simulink model "COSTEP_Exergy"  (R2024b)
settings: Solver=FixedStepAuto  StartTime=0.0  StopTime=25  FixedStep=1/3600  RelTol=1e-3
model workspace (MAT data in the model file):
  AD : Simulink.Parameter (value not decoded)
  AG : Simulink.Parameter (value not decoded)
  AH : Simulink.Parameter (value not decoded)
  AV : Simulink.Parameter (value not decoded)
  AVP : Simulink.Parameter (value not decoded)
  BCHL : Simulink.Parameter (value not decoded)
  BCHV : Simulink.Parameter (value not decoded)
  BD : Simulink.Parameter (value not decoded)
  BDIST : Simulink.Parameter (value not decoded)
  BG : Simulink.Parameter (value not decoded)
  BH : Simulink.Parameter (value not decoded)
  BVP : Simulink.Parameter (value not decoded)
  CD : Simulink.Parameter (value not decoded)
  CDIST : Simulink.Parameter (value not decoded)
  CG : Simulink.Parameter (value not decoded)
  CH : Simulink.Parameter (value not decoded)
  CVP : Simulink.Parameter (value not decoded)
  DDIST : Simulink.Parameter (value not decoded)
  DIST_CONST : Simulink.Parameter (value not decoded)
  ISV : Simulink.Parameter (value not decoded)
  TLAST : Simulink.Parameter (value not decoded)
  TNEXT : Simulink.Parameter (value not decoded)
  XMW : Simulink.Parameter (value not decoded)
  XNS : Simulink.Parameter (value not decoded)
  XNS2 : Simulink.Parameter (value not decoded)
  XNS3 : Simulink.Parameter (value not decoded)
  XNSADD : Simulink.Parameter (value not decoded)
  XNSE : Simulink.Parameter (value not decoded)
symbols that are objects in the model workspace (value not decoded): AD, AG, AH, AV, AVP, BD, BG, BH, BVP, CD, CG, CH, CVP, XMW, XNS, XNS2, XNS3, XNSE
undefined symbols (not defined in the file or in its folder): magnitude, msgbox, SETPT, XMEAS, XMV
libraries: mylib x403, dspindex x31
(part 13 of 13)

== system COSTEP_Exergy/Random number generator/Stream Measurements SMEAS Gas analysis1/If Action Subsystem3/Subsystem/Stream 5/Subsystem/TESUB6 XMNSEE ==
  G : Inport
  Process Noise I=1-12 G New : mylib/Process Noise I=1-12 G New  SystemSampleTime=-1  VariantActivationTime=update diagram  AllowFlexibleInterface=on  Latency=0  AutoFrameSizeCalculation=off
  XNSEE : Constant  Value=0.25
  XMNSEE : Outport  VectorParamsAs1DForOutWhenUnconnected=off
  G_NEW : Outport  Port=2  VectorParamsAs1DForOutWhenUnconnected=off
  wires:
  XNSEE/1 -> Process Noise I=1-12 G New/1
  Process Noise I=1-12 G New/1 -> XMNSEE/1
  G/1 -> Process Noise I=1-12 G New/2
  Process Noise I=1-12 G New/2 -> G_NEW/1

== system COSTEP_Exergy/Random number generator/Stream Measurements SMEAS Gas analysis1/If Action Subsystem3/Subsystem/Stream 5/Subsystem/TESUB6 XMNSEF ==
  G : Inport
  Process Noise I=1-12 G New : mylib/Process Noise I=1-12 G New  SystemSampleTime=-1  VariantActivationTime=update diagram  AllowFlexibleInterface=on  Latency=0  AutoFrameSizeCalculation=off
  XNSEF : Constant  Value=0.025
  XMNSEF : Outport  VectorParamsAs1DForOutWhenUnconnected=off
  G_NEW : Outport  Port=2  VectorParamsAs1DForOutWhenUnconnected=off
  wires:
  XNSEF/1 -> Process Noise I=1-12 G New/1
  Process Noise I=1-12 G New/1 -> XMNSEF/1
  G/1 -> Process Noise I=1-12 G New/2
  Process Noise I=1-12 G New/2 -> G_NEW/1

== system COSTEP_Exergy/Random number generator/Stream Measurements SMEAS Gas analysis1/If Action Subsystem3/Subsystem/Stream 5/Subsystem/TESUB6 XMNSEG ==
  G : Inport
  Process Noise I=1-12 G New : mylib/Process Noise I=1-12 G New  SystemSampleTime=-1  VariantActivationTime=update diagram  AllowFlexibleInterface=on  Latency=0  AutoFrameSizeCalculation=off
  XNSEG : Constant  Value=0.05
  XMNSEG : Outport  VectorParamsAs1DForOutWhenUnconnected=off
  G_NEW : Outport  Port=2  VectorParamsAs1DForOutWhenUnconnected=off
  wires:
  XNSEG/1 -> Process Noise I=1-12 G New/1
  Process Noise I=1-12 G New/1 -> XMNSEG/1
  G/1 -> Process Noise I=1-12 G New/2
  Process Noise I=1-12 G New/2 -> G_NEW/1

== system COSTEP_Exergy/Random number generator/Stream Measurements SMEAS Gas analysis1/If Action Subsystem3/Subsystem/Stream 5/Subsystem/TESUB6 XMNSEH ==
  G : Inport
  Process Noise I=1-12 G New : mylib/Process Noise I=1-12 G New  SystemSampleTime=-1  VariantActivationTime=update diagram  AllowFlexibleInterface=on  Latency=0  AutoFrameSizeCalculation=off
  XNSEH : Constant  Value=0.05
  XMNSEH : Outport  VectorParamsAs1DForOutWhenUnconnected=off
  G_NEW : Outport  Port=2  VectorParamsAs1DForOutWhenUnconnected=off
  wires:
  XNSEH/1 -> Process Noise I=1-12 G New/1
  Process Noise I=1-12 G New/1 -> XMNSEH/1
  G/1 -> Process Noise I=1-12 G New/2
  Process Noise I=1-12 G New/2 -> G_NEW/1

== system COSTEP_Exergy/Random number generator/Stream Measurements SMEAS Gas analysis1/If Action Subsystem3/Subsystem/Stream 6/Subsystem/TESUB6 XMNSEA ==
  G : Inport
  Process Noise I=1-12 G New : mylib/Process Noise I=1-12 G New  SystemSampleTime=-1  VariantActivationTime=update diagram  AllowFlexibleInterface=on  Latency=0  AutoFrameSizeCalculation=off
  XNSEA : Constant  Value=0.25
  XMNSEA : Outport  VectorParamsAs1DForOutWhenUnconnected=off
  G_NEW : Outport  Port=2  VectorParamsAs1DForOutWhenUnconnected=off
  wires:
  XNSEA/1 -> Process Noise I=1-12 G New/1
  Process Noise I=1-12 G New/1 -> XMNSEA/1
  G/1 -> Process Noise I=1-12 G New/2
  Process Noise I=1-12 G New/2 -> G_NEW/1

== system COSTEP_Exergy/Random number generator/Stream Measurements SMEAS Gas analysis1/If Action Subsystem3/Subsystem/Stream 6/Subsystem/TESUB6 XMNSEB ==
  G : Inport
  Process Noise I=1-12 G New : mylib/Process Noise I=1-12 G New  SystemSampleTime=-1  VariantActivationTime=update diagram  AllowFlexibleInterface=on  Latency=0  AutoFrameSizeCalculation=off
  XNSEB : Constant  Value=0.1
  XMNSEB : Outport  VectorParamsAs1DForOutWhenUnconnected=off
  G_NEW : Outport  Port=2  VectorParamsAs1DForOutWhenUnconnected=off
  wires:
  XNSEB/1 -> Process Noise I=1-12 G New/1
  Process Noise I=1-12 G New/1 -> XMNSEB/1
  G/1 -> Process Noise I=1-12 G New/2
  Process Noise I=1-12 G New/2 -> G_NEW/1

== system COSTEP_Exergy/Random number generator/Stream Measurements SMEAS Gas analysis1/If Action Subsystem3/Subsystem/Stream 6/Subsystem/TESUB6 XMNSEC ==
  G : Inport
  Process Noise I=1-12 G New : mylib/Process Noise I=1-12 G New  SystemSampleTime=-1  VariantActivationTime=update diagram  AllowFlexibleInterface=on  Latency=0  AutoFrameSizeCalculation=off
  XNSEC : Constant  Value=0.25
  XMNSEC : Outport  VectorParamsAs1DForOutWhenUnconnected=off
  G_NEW : Outport  Port=2  VectorParamsAs1DForOutWhenUnconnected=off
  wires:
  XNSEC/1 -> Process Noise I=1-12 G New/1
  Process Noise I=1-12 G New/1 -> XMNSEC/1
  G/1 -> Process Noise I=1-12 G New/2
  Process Noise I=1-12 G New/2 -> G_NEW/1

== system COSTEP_Exergy/Random number generator/Stream Measurements SMEAS Gas analysis1/If Action Subsystem3/Subsystem/Stream 6/Subsystem/TESUB6 XMNSED ==
  G : Inport
  Process Noise I=1-12 G New : mylib/Process Noise I=1-12 G New  SystemSampleTime=-1  VariantActivationTime=update diagram  AllowFlexibleInterface=on  Latency=0  AutoFrameSizeCalculation=off
  XNSED : Constant  Value=0.1
  XMNSED : Outport  VectorParamsAs1DForOutWhenUnconnected=off
  G_NEW : Outport  Port=2  VectorParamsAs1DForOutWhenUnconnected=off
  wires:
  XNSED/1 -> Process Noise I=1-12 G New/1
  Process Noise I=1-12 G New/1 -> XMNSED/1
  G/1 -> Process Noise I=1-12 G New/2
  Process Noise I=1-12 G New/2 -> G_NEW/1

== system COSTEP_Exergy/Random number generator/Stream Measurements SMEAS Gas analysis1/If Action Subsystem3/Subsystem/Stream 6/Subsystem/TESUB6 XMNSEE ==
  G : Inport
  Process Noise I=1-12 G New : mylib/Process Noise I=1-12 G New  SystemSampleTime=-1  VariantActivationTime=update diagram  AllowFlexibleInterface=on  Latency=0  AutoFrameSizeCalculation=off
  XNSEE : Constant  Value=0.25
  XMNSEE : Outport  VectorParamsAs1DForOutWhenUnconnected=off
  G_NEW : Outport  Port=2  VectorParamsAs1DForOutWhenUnconnected=off
  wires:
  XNSEE/1 -> Process Noise I=1-12 G New/1
  Process Noise I=1-12 G New/1 -> XMNSEE/1
  G/1 -> Process Noise I=1-12 G New/2
  Process Noise I=1-12 G New/2 -> G_NEW/1

== system COSTEP_Exergy/Random number generator/Stream Measurements SMEAS Gas analysis1/If Action Subsystem3/Subsystem/Stream 6/Subsystem/TESUB6 XMNSEF ==
  G : Inport
  Process Noise I=1-12 G New : mylib/Process Noise I=1-12 G New  SystemSampleTime=-1  VariantActivationTime=update diagram  AllowFlexibleInterface=on  Latency=0  AutoFrameSizeCalculation=off
  XNSEF : Constant  Value=0.025
  XMNSEF : Outport  VectorParamsAs1DForOutWhenUnconnected=off
  G_NEW : Outport  Port=2  VectorParamsAs1DForOutWhenUnconnected=off
  wires:
  XNSEF/1 -> Process Noise I=1-12 G New/1
  Process Noise I=1-12 G New/1 -> XMNSEF/1
  G/1 -> Process Noise I=1-12 G New/2
  Process Noise I=1-12 G New/2 -> G_NEW/1

== system COSTEP_Exergy/Random number generator/Stream Measurements SMEAS Gas analysis1/If Action Subsystem3/Subsystem/Stream 6/Subsystem/TESUB6 XMNSEG ==
  G : Inport
  Process Noise I=1-12 G New : mylib/Process Noise I=1-12 G New  SystemSampleTime=-1  VariantActivationTime=update diagram  AllowFlexibleInterface=on  Latency=0  AutoFrameSizeCalculation=off
  XNSEG : Constant  Value=0.05
  XMNSEG : Outport  VectorParamsAs1DForOutWhenUnconnected=off
  G_NEW : Outport  Port=2  VectorParamsAs1DForOutWhenUnconnected=off
  wires:
  XNSEG/1 -> Process Noise I=1-12 G New/1
  Process Noise I=1-12 G New/1 -> XMNSEG/1
  G/1 -> Process Noise I=1-12 G New/2
  Process Noise I=1-12 G New/2 -> G_NEW/1

== system COSTEP_Exergy/Random number generator/Stream Measurements SMEAS Gas analysis1/If Action Subsystem3/Subsystem/Stream 6/Subsystem/TESUB6 XMNSEH ==
  G : Inport
  Process Noise I=1-12 G New : mylib/Process Noise I=1-12 G New  SystemSampleTime=-1  VariantActivationTime=update diagram  AllowFlexibleInterface=on  Latency=0  AutoFrameSizeCalculation=off
  XNSEH : Constant  Value=0.05
  XMNSEH : Outport  VectorParamsAs1DForOutWhenUnconnected=off
  G_NEW : Outport  Port=2  VectorParamsAs1DForOutWhenUnconnected=off
  wires:
  XNSEH/1 -> Process Noise I=1-12 G New/1
  Process Noise I=1-12 G New/1 -> XMNSEH/1
  G/1 -> Process Noise I=1-12 G New/2
  Process Noise I=1-12 G New/2 -> G_NEW/1

== system COSTEP_Exergy/Random number generator/Stream Measurements SMEAS Gas analysis1/If Action Subsystem3/Subsystem/Stream 8/Subsystem/TESUB6 XMNSEA ==
  G : Inport
  Process Noise I=1-12 G New : mylib/Process Noise I=1-12 G New  SystemSampleTime=-1  VariantActivationTime=update diagram  AllowFlexibleInterface=on  Latency=0  AutoFrameSizeCalculation=off
  XNSEA : Constant  Value=0.25
  XMNSEA : Outport  VectorParamsAs1DForOutWhenUnconnected=off
  G_NEW : Outport  Port=2  VectorParamsAs1DForOutWhenUnconnected=off
  wires:
  XNSEA/1 -> Process Noise I=1-12 G New/1
  Process Noise I=1-12 G New/1 -> XMNSEA/1
  G/1 -> Process Noise I=1-12 G New/2
  Process Noise I=1-12 G New/2 -> G_NEW/1

== system COSTEP_Exergy/Random number generator/Stream Measurements SMEAS Gas analysis1/If Action Subsystem3/Subsystem/Stream 8/Subsystem/TESUB6 XMNSEB ==
  G : Inport
  Process Noise I=1-12 G New : mylib/Process Noise I=1-12 G New  SystemSampleTime=-1  VariantActivationTime=update diagram  AllowFlexibleInterface=on  Latency=0  AutoFrameSizeCalculation=off
  XNSEB : Constant  Value=0.1
  XMNSEB : Outport  VectorParamsAs1DForOutWhenUnconnected=off
  G_NEW : Outport  Port=2  VectorParamsAs1DForOutWhenUnconnected=off
  wires:
  XNSEB/1 -> Process Noise I=1-12 G New/1
  Process Noise I=1-12 G New/1 -> XMNSEB/1
  G/1 -> Process Noise I=1-12 G New/2
  Process Noise I=1-12 G New/2 -> G_NEW/1

== system COSTEP_Exergy/Random number generator/Stream Measurements SMEAS Gas analysis1/If Action Subsystem3/Subsystem/Stream 8/Subsystem/TESUB6 XMNSEC ==
  G : Inport
  Process Noise I=1-12 G New : mylib/Process Noise I=1-12 G New  SystemSampleTime=-1  VariantActivationTime=update diagram  AllowFlexibleInterface=on  Latency=0  AutoFrameSizeCalculation=off
  XNSEC : Constant  Value=0.25
  XMNSEC : Outport  VectorParamsAs1DForOutWhenUnconnected=off
  G_NEW : Outport  Port=2  VectorParamsAs1DForOutWhenUnconnected=off
  wires:
  XNSEC/1 -> Process Noise I=1-12 G New/1
  Process Noise I=1-12 G New/1 -> XMNSEC/1
  G/1 -> Process Noise I=1-12 G New/2
  Process Noise I=1-12 G New/2 -> G_NEW/1

== system COSTEP_Exergy/Random number generator/Stream Measurements SMEAS Gas analysis1/If Action Subsystem3/Subsystem/Stream 8/Subsystem/TESUB6 XMNSED ==
  G : Inport
  Process Noise I=1-12 G New : mylib/Process Noise I=1-12 G New  SystemSampleTime=-1  VariantActivationTime=update diagram  AllowFlexibleInterface=on  Latency=0  AutoFrameSizeCalculation=off
  XNSED : Constant  Value=0.1
  XMNSED : Outport  VectorParamsAs1DForOutWhenUnconnected=off
  G_NEW : Outport  Port=2  VectorParamsAs1DForOutWhenUnconnected=off
  wires:
  XNSED/1 -> Process Noise I=1-12 G New/1
  Process Noise I=1-12 G New/1 -> XMNSED/1
  G/1 -> Process Noise I=1-12 G New/2
  Process Noise I=1-12 G New/2 -> G_NEW/1

== system COSTEP_Exergy/Random number generator/Stream Measurements SMEAS Gas analysis1/If Action Subsystem3/Subsystem/Stream 8/Subsystem/TESUB6 XMNSEE ==
  G : Inport
  Process Noise I=1-12 G New : mylib/Process Noise I=1-12 G New  SystemSampleTime=-1  VariantActivationTime=update diagram  AllowFlexibleInterface=on  Latency=0  AutoFrameSizeCalculation=off
  XNSEE : Constant  Value=0.25
  XMNSEE : Outport  VectorParamsAs1DForOutWhenUnconnected=off
  G_NEW : Outport  Port=2  VectorParamsAs1DForOutWhenUnconnected=off
  wires:
  XNSEE/1 -> Process Noise I=1-12 G New/1
  Process Noise I=1-12 G New/1 -> XMNSEE/1
  G/1 -> Process Noise I=1-12 G New/2
  Process Noise I=1-12 G New/2 -> G_NEW/1

== system COSTEP_Exergy/Random number generator/Stream Measurements SMEAS Gas analysis1/If Action Subsystem3/Subsystem/Stream 8/Subsystem/TESUB6 XMNSEF ==
  G : Inport
  Process Noise I=1-12 G New : mylib/Process Noise I=1-12 G New  SystemSampleTime=-1  VariantActivationTime=update diagram  AllowFlexibleInterface=on  Latency=0  AutoFrameSizeCalculation=off
  XNSEF : Constant  Value=0.025
  XMNSEF : Outport  VectorParamsAs1DForOutWhenUnconnected=off
  G_NEW : Outport  Port=2  VectorParamsAs1DForOutWhenUnconnected=off
  wires:
  XNSEF/1 -> Process Noise I=1-12 G New/1
  Process Noise I=1-12 G New/1 -> XMNSEF/1
  G/1 -> Process Noise I=1-12 G New/2
  Process Noise I=1-12 G New/2 -> G_NEW/1

== system COSTEP_Exergy/Random number generator/Stream Measurements SMEAS Gas analysis1/If Action Subsystem3/Subsystem/Stream 8/Subsystem/TESUB6 XMNSEG ==
  G : Inport
  Process Noise I=1-12 G New : mylib/Process Noise I=1-12 G New  SystemSampleTime=-1  VariantActivationTime=update diagram  AllowFlexibleInterface=on  Latency=0  AutoFrameSizeCalculation=off
  XNSEG : Constant  Value=0.05
  XMNSEG : Outport  VectorParamsAs1DForOutWhenUnconnected=off
  G_NEW : Outport  Port=2  VectorParamsAs1DForOutWhenUnconnected=off
  wires:
  XNSEG/1 -> Process Noise I=1-12 G New/1
  Process Noise I=1-12 G New/1 -> XMNSEG/1
  G/1 -> Process Noise I=1-12 G New/2
  Process Noise I=1-12 G New/2 -> G_NEW/1

== system COSTEP_Exergy/Random number generator/Stream Measurements SMEAS Gas analysis1/If Action Subsystem3/Subsystem/Stream 8/Subsystem/TESUB6 XMNSEH ==
  G : Inport
  Process Noise I=1-12 G New : mylib/Process Noise I=1-12 G New  SystemSampleTime=-1  VariantActivationTime=update diagram  AllowFlexibleInterface=on  Latency=0  AutoFrameSizeCalculation=off
  XNSEH : Constant  Value=0.05
  XMNSEH : Outport  VectorParamsAs1DForOutWhenUnconnected=off
  G_NEW : Outport  Port=2  VectorParamsAs1DForOutWhenUnconnected=off
  wires:
  XNSEH/1 -> Process Noise I=1-12 G New/1
  Process Noise I=1-12 G New/1 -> XMNSEH/1
  G/1 -> Process Noise I=1-12 G New/2
  Process Noise I=1-12 G New/2 -> G_NEW/1

== system COSTEP_Exergy/Random number generator/Stream Measurements SMEAS Gas analysis1/If Action Subsystem3/Subsystem/Stream 9/Subsystem/TESUB6 XMNSEA ==
  G : Inport
  Process Noise I=1-12 G New : mylib/Process Noise I=1-12 G New  SystemSampleTime=-1  VariantActivationTime=update diagram  AllowFlexibleInterface=on  Latency=0  AutoFrameSizeCalculation=off
  XNSEA : Constant  Value=0.25
  XMNSEA : Outport  VectorParamsAs1DForOutWhenUnconnected=off
  G_NEW : Outport  Port=2  VectorParamsAs1DForOutWhenUnconnected=off
  wires:
  XNSEA/1 -> Process Noise I=1-12 G New/1
  Process Noise I=1-12 G New/1 -> XMNSEA/1
  G/1 -> Process Noise I=1-12 G New/2
  Process Noise I=1-12 G New/2 -> G_NEW/1

== system COSTEP_Exergy/Random number generator/Stream Measurements SMEAS Gas analysis1/If Action Subsystem3/Subsystem/Stream 9/Subsystem/TESUB6 XMNSEB ==
  G : Inport
  Process Noise I=1-12 G New : mylib/Process Noise I=1-12 G New  SystemSampleTime=-1  VariantActivationTime=update diagram  AllowFlexibleInterface=on  Latency=0  AutoFrameSizeCalculation=off
  XNSEB : Constant  Value=0.1
  XMNSEB : Outport  VectorParamsAs1DForOutWhenUnconnected=off
  G_NEW : Outport  Port=2  VectorParamsAs1DForOutWhenUnconnected=off
  wires:
  XNSEB/1 -> Process Noise I=1-12 G New/1
  Process Noise I=1-12 G New/1 -> XMNSEB/1
  G/1 -> Process Noise I=1-12 G New/2
  Process Noise I=1-12 G New/2 -> G_NEW/1

== system COSTEP_Exergy/Random number generator/Stream Measurements SMEAS Gas analysis1/If Action Subsystem3/Subsystem/Stream 9/Subsystem/TESUB6 XMNSEC ==
  G : Inport
  Process Noise I=1-12 G New : mylib/Process Noise I=1-12 G New  SystemSampleTime=-1  VariantActivationTime=update diagram  AllowFlexibleInterface=on  Latency=0  AutoFrameSizeCalculation=off
  XNSEC : Constant  Value=0.25
  XMNSEC : Outport  VectorParamsAs1DForOutWhenUnconnected=off
  G_NEW : Outport  Port=2  VectorParamsAs1DForOutWhenUnconnected=off
  wires:
  XNSEC/1 -> Process Noise I=1-12 G New/1
  Process Noise I=1-12 G New/1 -> XMNSEC/1
  G/1 -> Process Noise I=1-12 G New/2
  Process Noise I=1-12 G New/2 -> G_NEW/1

== system COSTEP_Exergy/Random number generator/Stream Measurements SMEAS Gas analysis1/If Action Subsystem3/Subsystem/Stream 9/Subsystem/TESUB6 XMNSED ==
  G : Inport
  Process Noise I=1-12 G New : mylib/Process Noise I=1-12 G New  SystemSampleTime=-1  VariantActivationTime=update diagram  AllowFlexibleInterface=on  Latency=0  AutoFrameSizeCalculation=off
  XNSED : Constant  Value=0.1
  XMNSED : Outport  VectorParamsAs1DForOutWhenUnconnected=off
  G_NEW : Outport  Port=2  VectorParamsAs1DForOutWhenUnconnected=off
  wires:
  XNSED/1 -> Process Noise I=1-12 G New/1
  Process Noise I=1-12 G New/1 -> XMNSED/1
  G/1 -> Process Noise I=1-12 G New/2
  Process Noise I=1-12 G New/2 -> G_NEW/1

== system COSTEP_Exergy/Random number generator/Stream Measurements SMEAS Gas analysis1/If Action Subsystem3/Subsystem/Stream 9/Subsystem/TESUB6 XMNSEE ==
  G : Inport
  Process Noise I=1-12 G New : mylib/Process Noise I=1-12 G New  SystemSampleTime=-1  VariantActivationTime=update diagram  AllowFlexibleInterface=on  Latency=0  AutoFrameSizeCalculation=off
  XNSEE : Constant  Value=0.25
  XMNSEE : Outport  VectorParamsAs1DForOutWhenUnconnected=off
  G_NEW : Outport  Port=2  VectorParamsAs1DForOutWhenUnconnected=off
  wires:
  XNSEE/1 -> Process Noise I=1-12 G New/1
  Process Noise I=1-12 G New/1 -> XMNSEE/1
  G/1 -> Process Noise I=1-12 G New/2
  Process Noise I=1-12 G New/2 -> G_NEW/1

== system COSTEP_Exergy/Random number generator/Stream Measurements SMEAS Gas analysis1/If Action Subsystem3/Subsystem/Stream 9/Subsystem/TESUB6 XMNSEF ==
  G : Inport
  Process Noise I=1-12 G New : mylib/Process Noise I=1-12 G New  SystemSampleTime=-1  VariantActivationTime=update diagram  AllowFlexibleInterface=on  Latency=0  AutoFrameSizeCalculation=off
  XNSEF : Constant  Value=0.025
  XMNSEF : Outport  VectorParamsAs1DForOutWhenUnconnected=off
  G_NEW : Outport  Port=2  VectorParamsAs1DForOutWhenUnconnected=off
  wires:
  XNSEF/1 -> Process Noise I=1-12 G New/1
  Process Noise I=1-12 G New/1 -> XMNSEF/1
  G/1 -> Process Noise I=1-12 G New/2
  Process Noise I=1-12 G New/2 -> G_NEW/1

== system COSTEP_Exergy/Random number generator/Stream Measurements SMEAS Gas analysis1/If Action Subsystem3/Subsystem/Stream 9/Subsystem/TESUB6 XMNSEG ==
  G : Inport
  Process Noise I=1-12 G New : mylib/Process Noise I=1-12 G New  SystemSampleTime=-1  VariantActivationTime=update diagram  AllowFlexibleInterface=on  Latency=0  AutoFrameSizeCalculation=off
  XNSEG : Constant  Value=0.05
  XMNSEG : Outport  VectorParamsAs1DForOutWhenUnconnected=off
  G_NEW : Outport  Port=2  VectorParamsAs1DForOutWhenUnconnected=off
  wires:
  XNSEG/1 -> Process Noise I=1-12 G New/1
  Process Noise I=1-12 G New/1 -> XMNSEG/1
  G/1 -> Process Noise I=1-12 G New/2
  Process Noise I=1-12 G New/2 -> G_NEW/1

== system COSTEP_Exergy/Random number generator/Stream Measurements SMEAS Gas analysis1/If Action Subsystem3/Subsystem/Stream 9/Subsystem/TESUB6 XMNSEH ==
  G : Inport
  Process Noise I=1-12 G New : mylib/Process Noise I=1-12 G New  SystemSampleTime=-1  VariantActivationTime=update diagram  AllowFlexibleInterface=on  Latency=0  AutoFrameSizeCalculation=off
  XNSEH : Constant  Value=0.05
  XMNSEH : Outport  VectorParamsAs1DForOutWhenUnconnected=off
  G_NEW : Outport  Port=2  VectorParamsAs1DForOutWhenUnconnected=off
  wires:
  XNSEH/1 -> Process Noise I=1-12 G New/1
  Process Noise I=1-12 G New/1 -> XMNSEH/1
  G/1 -> Process Noise I=1-12 G New/2
  Process Noise I=1-12 G New/2 -> G_NEW/1

== system COSTEP_Exergy/Random number generator/Stream Measurements SMEAS Product analysis1/If Action Subsystem3/Subsystem/Subsystem1/Subsystem/TESUB6 XMNSED ==
  G : Inport
  Process Noise I=1-12 G New : mylib/Process Noise I=1-12 G New  SystemSampleTime=-1  VariantActivationTime=update diagram  AllowFlexibleInterface=on  Latency=0  AutoFrameSizeCalculation=off
  XNS(37) : Constant  Value=0.01
  XMNS : Outport  VectorParamsAs1DForOutWhenUnconnected=off
  G_NEW : Outport  Port=2  VectorParamsAs1DForOutWhenUnconnected=off
  wires:
  XNS(37)/1 -> Process Noise I=1-12 G New/1
  Process Noise I=1-12 G New/1 -> XMNS/1
  G/1 -> Process Noise I=1-12 G New/2
  Process Noise I=1-12 G New/2 -> G_NEW/1

== system COSTEP_Exergy/Random number generator/Stream Measurements SMEAS Product analysis1/If Action Subsystem3/Subsystem/Subsystem1/Subsystem/TESUB6 XMNSEE ==
  G : Inport
  Process Noise I=1-12 G New : mylib/Process Noise I=1-12 G New  SystemSampleTime=-1  VariantActivationTime=update diagram  AllowFlexibleInterface=on  Latency=0  AutoFrameSizeCalculation=off
  XNS(38) : Constant  Value=0.01
  XMNS : Outport  VectorParamsAs1DForOutWhenUnconnected=off
  G_NEW : Outport  Port=2  VectorParamsAs1DForOutWhenUnconnected=off
  wires:
  XNS(38)/1 -> Process Noise I=1-12 G New/1
  Process Noise I=1-12 G New/1 -> XMNS/1
  G/1 -> Process Noise I=1-12 G New/2
  Process Noise I=1-12 G New/2 -> G_NEW/1

== system COSTEP_Exergy/Random number generator/Stream Measurements SMEAS Product analysis1/If Action Subsystem3/Subsystem/Subsystem1/Subsystem/TESUB6 XMNSEF ==
  G : Inport
  Process Noise I=1-12 G New : mylib/Process Noise I=1-12 G New  SystemSampleTime=-1  VariantActivationTime=update diagram  AllowFlexibleInterface=on  Latency=0  AutoFrameSizeCalculation=off
  XNS(39) : Constant  Value=0.01
  XMNS : Outport  VectorParamsAs1DForOutWhenUnconnected=off
  G_NEW : Outport  Port=2  VectorParamsAs1DForOutWhenUnconnected=off
  wires:
  XNS(39)/1 -> Process Noise I=1-12 G New/1
  Process Noise I=1-12 G New/1 -> XMNS/1
  G/1 -> Process Noise I=1-12 G New/2
  Process Noise I=1-12 G New/2 -> G_NEW/1

== system COSTEP_Exergy/Random number generator/Stream Measurements SMEAS Product analysis1/If Action Subsystem3/Subsystem/Subsystem1/Subsystem/TESUB6 XMNSEG ==
  G : Inport
  Process Noise I=1-12 G New : mylib/Process Noise I=1-12 G New  SystemSampleTime=-1  VariantActivationTime=update diagram  AllowFlexibleInterface=on  Latency=0  AutoFrameSizeCalculation=off
  XNS(40) : Constant  Value=0.5
  XMNS : Outport  VectorParamsAs1DForOutWhenUnconnected=off
  G_NEW : Outport  Port=2  VectorParamsAs1DForOutWhenUnconnected=off
  wires:
  XNS(40)/1 -> Process Noise I=1-12 G New/1
  Process Noise I=1-12 G New/1 -> XMNS/1
  G/1 -> Process Noise I=1-12 G New/2
  Process Noise I=1-12 G New/2 -> G_NEW/1

== system COSTEP_Exergy/Random number generator/Stream Measurements SMEAS Product analysis1/If Action Subsystem3/Subsystem/Subsystem1/Subsystem/TESUB6 XMNSEH ==
  G : Inport
  Process Noise I=1-12 G New : mylib/Process Noise I=1-12 G New  SystemSampleTime=-1  VariantActivationTime=update diagram  AllowFlexibleInterface=on  Latency=0  AutoFrameSizeCalculation=off
  XNS(41) : Constant  Value=0.5
  XMNS : Outport  VectorParamsAs1DForOutWhenUnconnected=off
  G_NEW : Outport  Port=2  VectorParamsAs1DForOutWhenUnconnected=off
  wires:
  XNS(41)/1 -> Process Noise I=1-12 G New/1
  Process Noise I=1-12 G New/1 -> XMNS/1
  G/1 -> Process Noise I=1-12 G New/2
  Process Noise I=1-12 G New/2 -> G_NEW/1

== system COSTEP_Exergy/Random number generator/Stream Measurements SMEAS Product analysis1/If Action Subsystem3/Subsystem/Subsystem2/Subsystem/TESUB6 XMNSED ==
  G : Inport
  Process Noise I=1-12 G New : mylib/Process Noise I=1-12 G New  SystemSampleTime=-1  VariantActivationTime=update diagram  AllowFlexibleInterface=on  Latency=0  AutoFrameSizeCalculation=off
  XNS(37) : Constant  Value=0.01
  XMNS : Outport  VectorParamsAs1DForOutWhenUnconnected=off
  G_NEW : Outport  Port=2  VectorParamsAs1DForOutWhenUnconnected=off
  wires:
  XNS(37)/1 -> Process Noise I=1-12 G New/1
  Process Noise I=1-12 G New/1 -> XMNS/1
  G/1 -> Process Noise I=1-12 G New/2
  Process Noise I=1-12 G New/2 -> G_NEW/1

== system COSTEP_Exergy/Random number generator/Stream Measurements SMEAS Product analysis1/If Action Subsystem3/Subsystem/Subsystem2/Subsystem/TESUB6 XMNSEE ==
  G : Inport
  Process Noise I=1-12 G New : mylib/Process Noise I=1-12 G New  SystemSampleTime=-1  VariantActivationTime=update diagram  AllowFlexibleInterface=on  Latency=0  AutoFrameSizeCalculation=off
  XNS(38) : Constant  Value=0.01
  XMNS : Outport  VectorParamsAs1DForOutWhenUnconnected=off
  G_NEW : Outport  Port=2  VectorParamsAs1DForOutWhenUnconnected=off
  wires:
  XNS(38)/1 -> Process Noise I=1-12 G New/1
  Process Noise I=1-12 G New/1 -> XMNS/1
  G/1 -> Process Noise I=1-12 G New/2
  Process Noise I=1-12 G New/2 -> G_NEW/1

== system COSTEP_Exergy/Random number generator/Stream Measurements SMEAS Product analysis1/If Action Subsystem3/Subsystem/Subsystem2/Subsystem/TESUB6 XMNSEF ==
  G : Inport
  Process Noise I=1-12 G New : mylib/Process Noise I=1-12 G New  SystemSampleTime=-1  VariantActivationTime=update diagram  AllowFlexibleInterface=on  Latency=0  AutoFrameSizeCalculation=off
  XNS(39) : Constant  Value=0.01
  XMNS : Outport  VectorParamsAs1DForOutWhenUnconnected=off
  G_NEW : Outport  Port=2  VectorParamsAs1DForOutWhenUnconnected=off
  wires:
  XNS(39)/1 -> Process Noise I=1-12 G New/1
  Process Noise I=1-12 G New/1 -> XMNS/1
  G/1 -> Process Noise I=1-12 G New/2
  Process Noise I=1-12 G New/2 -> G_NEW/1

== system COSTEP_Exergy/Random number generator/Stream Measurements SMEAS Product analysis1/If Action Subsystem3/Subsystem/Subsystem2/Subsystem/TESUB6 XMNSEG ==
  G : Inport
  Process Noise I=1-12 G New : mylib/Process Noise I=1-12 G New  SystemSampleTime=-1  VariantActivationTime=update diagram  AllowFlexibleInterface=on  Latency=0  AutoFrameSizeCalculation=off
  XNS(40) : Constant  Value=0.5
  XMNS : Outport  VectorParamsAs1DForOutWhenUnconnected=off
  G_NEW : Outport  Port=2  VectorParamsAs1DForOutWhenUnconnected=off
  wires:
  XNS(40)/1 -> Process Noise I=1-12 G New/1
  Process Noise I=1-12 G New/1 -> XMNS/1
  G/1 -> Process Noise I=1-12 G New/2
  Process Noise I=1-12 G New/2 -> G_NEW/1

== system COSTEP_Exergy/Random number generator/Stream Measurements SMEAS Product analysis1/If Action Subsystem3/Subsystem/Subsystem2/Subsystem/TESUB6 XMNSEH ==
  G : Inport
  Process Noise I=1-12 G New : mylib/Process Noise I=1-12 G New  SystemSampleTime=-1  VariantActivationTime=update diagram  AllowFlexibleInterface=on  Latency=0  AutoFrameSizeCalculation=off
  XNS(41) : Constant  Value=0.5
  XMNS : Outport  VectorParamsAs1DForOutWhenUnconnected=off
  G_NEW : Outport  Port=2  VectorParamsAs1DForOutWhenUnconnected=off
  wires:
  XNS(41)/1 -> Process Noise I=1-12 G New/1
  Process Noise I=1-12 G New/1 -> XMNS/1
  G/1 -> Process Noise I=1-12 G New/2
  Process Noise I=1-12 G New/2 -> G_NEW/1

== matlab function COSTEP_Exergy/Stream Measurements/Subsystem6/Separator recycle stream (after compressor)/Temperature measurement in C/TST(9) Temperature of Stream °C /MATLAB Function ==
  data: AH input; TST output; BH input; CH input; AG input; BG input; CG input; AV input; XMW input; XLR input; HST input; ITY input; TST input
function TST  = TempLoop(AH,BH,CH,AG,BG,CG,AV,XMW,XLR,HST,ITY,TST)
  
Z = XLR;
T = TST;
H = HST;
TIN=T;

for J = 1:100
	
	if ITY == 0
    	HTEST = 0;
		for I = 1:8
      		HI = T * (AH(I,1) + BH(I,1) * T / 2 + CH(I,1) * T^2 / 3);
      		HI = 1.8 * HI;
      		HTEST = HTEST + Z(I,1) * XMW(I,1) * HI;
		end
	else
      	HTEST = 0;
		for I = 1:8 
      		HI = T * (AG(I,1) + BG(I,1) * T / 2 + CG(I,1) * T^2 / 3);
      		HI = 1.8 * HI;
      		HI = HI + AV(I,1);
      		HTEST = HTEST + Z(I,1) * XMW(I,1) * HI;
		end
    end
        if ITY == 2
         	R1 = 3.57696 / 1000000;
        	HTEST = HTEST - R1 * (T + 273.15);
    	end
		
    ERR = HTEST - H;
	
	if ITY == 0
      	DH = 0.0;
    	for I = 1:8
      		DHI = AH(I,1) + BH(I,1) * T + CH(I,1) * T^2;
      		DHI = 1.8 * DHI;
      		DH = DH + Z(I,1) * XMW(I,1) * DHI;
		end
	else
      	DH=0.0;
    	for I = 1:8
      		DHI = AG(I,1) + BG(I,1) * T + CG(I,1) * T^2;
      		DHI = 1.8 * DHI;
      		DH = DH + Z(I,1) * XMW(I,1) * DHI;
		end
    end
    
    if ITY == 2
      	R3 = 3.57696/1000000;
     	DH = DH - R3;
 	end
	
    DT = -ERR / DH;
    T = T + DT;
  	if abs(DT) < 1*10^(-12)
    	break
  	end
  	if J == 100
  		T = TIN;
  	end
end
TST = T;

== matlab function COSTEP_Exergy/Stream Measurements/Subsystem6/Condenser product stream/Subsystem/TST(8a) Temperature of Stream °C /MATLAB Function ==
  data: AH input; TST output; BH input; CH input; AG input; BG input; CG input; AV input; XMW input; XLR input; HST input; ITY input; TST input
function TST  = TempLoop(AH,BH,CH,AG,BG,CG,AV,XMW,XLR,HST,ITY,TST)
  
Z = XLR;
T = TST;
H = HST;
TIN=T;

for J = 1:100
	
	if ITY == 0
    	HTEST = 0;
		for I = 1:8
      		HI = T * (AH(I,1) + BH(I,1) * T / 2 + CH(I,1) * T^2 / 3);
      		HI = 1.8 * HI;
      		HTEST = HTEST + Z(I,1) * XMW(I,1) * HI;
		end
	else
      	HTEST = 0;
		for I = 1:8 
      		HI = T * (AG(I,1) + BG(I,1) * T / 2 + CG(I,1) * T^2 / 3);
      		HI = 1.8 * HI;
      		HI = HI + AV(I,1);
      		HTEST = HTEST + Z(I,1) * XMW(I,1) * HI;
		end
    end
        if ITY == 2
         	R1 = 3.57696 / 1000000;
        	HTEST = HTEST - R1 * (T + 273.15);
    	end
		
    ERR = HTEST - H;
	
	if ITY == 0
      	DH = 0.0;
    	for I = 1:8
      		DHI = AH(I,1) + BH(I,1) * T + CH(I,1) * T^2;
      		DHI = 1.8 * DHI;
      		DH = DH + Z(I,1) * XMW(I,1) * DHI;
		end
	else
      	DH=0.0;
    	for I = 1:8
      		DHI = AG(I,1) + BG(I,1) * T + CG(I,1) * T^2;
      		DHI = 1.8 * DHI;
      		DH = DH + Z(I,1) * XMW(I,1) * DHI;
		end
    end
    
    if ITY == 2
      	R3 = 3.57696/1000000;
     	DH = DH - R3;
 	end
	
    DT = -ERR / DH;
    T = T + DT;
  	if abs(DT) < 1*10^(-12)
    	break
  	end
  	if J == 100
  		T = TIN;
  	end
end
TST = T;

== matlab function COSTEP_Exergy/Mode Selection/MATLAB Function ==
  data: M input; M_out output
function M_out = checkM(M)
    M_out = zeros(1, 1);
    coder.extrinsic("evalin")
    % Lets first check if "M" exists in the workspace form
    % Auto_run_COSTEP.m
    ise = evalin('base', 'exist(''M'',''var'') == 1');
    if ise 
        M_out = evalin('base', 'M');
    else
        M_out = M;
    end
end

== matlab function COSTEP_Exergy/Disturbances/MATLAB Function ==
  data: IDV input; IDV_out output
function IDV_out = checkIDV(IDV)
    IDV_out = zeros(28, 1);
    coder.extrinsic("evalin")
    % Lets first check if "IDV" exists in the workspace form
    % Auto_run_COSTEP.m
    ise = evalin('base', 'exist(''IDV'',''var'') == 1');
    if ise 
        IDV_out = evalin('base', 'IDV');
    else
        IDV_out = IDV;
    end
end

== matlab function COSTEP_Exergy/Random number generator/Process Measurements XMEAS(I) I=1-22/MATLAB Function ==
  data: XNS input; G output; G input; ISD input; Time input; XMNS output
function [G,XMNS] = ProcessNoise(XNS,G,ISD,Time)

XNS = XNS(1:22, :); % Select only the first 22 rows
X=zeros(22,1);
RN=zeros(22*12+1,1);
RN(1,1)=G;
TESUB7 = zeros(12,22);

if Time > 0.0 && ISD == 0

    for I=1:22
        
    TESUB7_value = zeros(1,22);
    
        for It =1:12
    
            RN((12*I-11+It),1) = mod(RN((12*I-11+It-1),1) * 9228907,4294967296);
                if It >= 0
                    TESUB7_value(I) = RN((12*I-11+It),1) / 4294967296;
                else
                    TESUB7_value(I) = 2 * RN((12*I-11+It),1) / 4294967296 - 1;
                end
            TESUB7(It,I)=TESUB7_value(I); 
            X(I) = X(I) + TESUB7(It,I);
        end 
    
        X(I) = (X(I) - 6) * XNS(I,1);
        XMNS = X;
    end 
    
    G = RN(end);
    
else
    XMNS = zeros(22,1);
    G = RN(1,1);
end

== matlab function COSTEP_Exergy/Random number generator/Process Measurements XMEAS(I) I=23-36/MATLAB Function ==
  data: XNS input; G output; G input; XMNS output; TIME input; XMNS input
function [G,XMNS] = ProcessNoise(XNS,G,TIME, XMNS)

X =zeros(14,1);
RN=zeros(14*12+1,1);
RN(1,1)=G;
TESUB7 = zeros(12,14);
TGAS = 0.1*3600;
T = TIME*3600;
Test = round(mod(T,TGAS));
XN=XMNS;

if TIME>0 & Test==0 | Test==360 ;

    for I=1:14
        
    TESUB7_value = zeros(1,14);
    
    for It =1:12
    
            RN((12*I-11+It),1) = mod(RN((12*I-11+It-1),1) * 9228907,4294967296);
                if It >= 0
                    TESUB7_value(I) = RN((12*I-11+It),1) / 4294967296;
                else
                    TESUB7_value(I) = 2 * RN((12*I-11+It),1) / 4294967296 - 1;
                end
            TESUB7(It,I)=TESUB7_value(I); 
            X(I) = X(I) + TESUB7(It,I);
    end 
    
        X(I) = (X(I) - 6) * XNS(I,1);
        
    end
    
    XMNS = X;
    G = RN(end);

else
    
    XMNS = XN;
    G = RN(1,1);
    
end

== matlab function COSTEP_Exergy/Random number generator/Process Measurements XMEAS(I) I=37-41/MATLAB Function ==
  data: XNS input; G output; G input; XMNS output; TIME input; XMNS input
function [G,XMNS] = ProcessNoise(XNS,G,TIME, XMNS)

X =zeros(5,1);
RN=zeros(5*12+1,1);
RN(1,1)=G;
TESUB7 = zeros(12,5);
TPROD = 0.25*3600;
T = TIME*3600;
Test = round(mod(T,TPROD));
XN=XMNS;

if TIME>0 & Test==0 | Test == 900;

    for I=1:5
        
    TESUB7_value = zeros(1,5);
    
    for It =1:12
    
            RN((12*I-11+It),1) = mod(RN((12*I-11+It-1),1) * 9228907,4294967296);
                if It >= 0
                    TESUB7_value(I) = RN((12*I-11+It),1) / 4294967296;
                else
                    TESUB7_value(I) = 2 * RN((12*I-11+It),1) / 4294967296 - 1;
                end
            TESUB7(It,I)=TESUB7_value(I); 
            X(I) = X(I) + TESUB7(It,I);
    end 
    
        X(I) = (X(I) - 6) * XNS(I,1);
        
    end 
    XMNS = X;
    G = RN(end);
    
else
    
    XMNS = XN;
    G = RN(1,1);
    
end

== matlab function COSTEP_Exergy/Random number generator/Stream Measurements SMEAS1/MATLAB Function ==
  data: XNSE input; GE output; GE input; ISD input; Time input; XMNSE output
function [GE,XMNSE] = ProcessNoise(XNSE,GE,ISD,Time)

X =zeros(24,1);
RN=zeros(24*12+1,1);
RN(1,1)=GE;
TESUB7 = zeros(12,24);

if Time > 0.0 && ISD == 0

    for I=1:24
        
    TESUB7_value = zeros(1,24);
    
        for It =1:12
    
            RN((12*I-11+It),1) = mod(RN((12*I-11+It-1),1) * 9228907,4294967296);
                if It >= 0
                    TESUB7_value(I) = RN((12*I-11+It),1) / 4294967296;
                else
                    TESUB7_value(I) = 2 * RN((12*I-11+It),1) / 4294967296 - 1;
                end
            TESUB7(It,I)=TESUB7_value(I); 
            X(I) = X(I) + TESUB7(It,I);
        end 
    
        X(I) = (X(I) - 6) * XNSE(I,1);
        XMNSE = X;
    end 
    
    GE = RN(end);
    
else
    XMNSE = zeros(24,1);
    GE = RN(1,1);
end

== matlab function COSTEP_Exergy/Separator/TCS Initial Temperature in Separator °C /MATLAB Function ==
  data: AH input; TCS output; BH input; CH input; AG input; BG input; CG input; AV input; XMW input; XLS input; ETS input; UTLS input; ITY input; TCS input
function TCS  = TempLoop(AH,BH,CH,AG,BG,CG,AV,XMW,XLS,ETS,UTLS,ITY,TCS)

ESS = ETS/UTLS;
     
Z = XLS;
T = TCS;
H = ESS;
TIN=T;

for J = 1:100
	
	if ITY == 0
    	HTEST = 0;
		for I = 1:8
      		HI = T * (AH(I,1) + BH(I,1) * T / 2 + CH(I,1) * T^2 / 3);
      		HI = 1.8 * HI;
      		HTEST = HTEST + Z(I,1) * XMW(I,1) * HI;
		end
	else
      	HTEST = 0;
		for I = 1:8 
      		HI = T * (AG(I,1) + BG(I,1) * T / 2 + CG(I,1) * T^2 / 3);
      		HI = 1.8 * HI;
      		HI = HI + AV(I,1);
      		HTEST = HTEST + Z(I,1) * XMW(I,1) * HI;
		end
    end
        if ITY == 2
         	R1 = 3.57696 / 1000000;
        	HTEST = HTEST - R1 * (T + 273.15);
    	end
		
    ERR = HTEST - H;
	
	if ITY == 0
      	DH = 0.0;
    	for I = 1:8
      		DHI = AH(I,1) + BH(I,1) * T + CH(I,1) * T^2;
      		DHI = 1.8 * DHI;
      		DH = DH + Z(I,1) * XMW(I,1) * DHI;
		end
	else
      	DH=0.0;
    	for I = 1:8
      		DHI = AG(I,1) + BG(I,1) * T + CG(I,1) * T^2;
      		DHI = 1.8 * DHI;
      		DH = DH + Z(I,1) * XMW(I,1) * DHI;
		end
    end
    
    if ITY == 2
      	R3 = 3.57696/1000000;
     	DH = DH - R3;
 	end
	
    DT = -ERR / DH;
    T = T + DT;
  	if abs(DT) < 1*10^(-12)
    	break
  	end
  	if J == 100
  		T = TIN;
  	end
end
TCS = T;

== matlab function COSTEP_Exergy/Reactor/TCR Initial Temperature in Reactor °C /MATLAB Function ==
  data: AH input; TCR output; BH input; CH input; AG input; BG input; CG input; AV input; XMW input; XLR input; ETR input; UTLR input; ITY input; TCR input
function TCR  = TempLoop(AH,BH,CH,AG,BG,CG,AV,XMW,XLR,ETR,UTLR,ITY,TCR)

ESR = ETR/UTLR;
     
Z = XLR;
T = TCR;
H = ESR;
TIN=T;

for J = 1:100
	
	if ITY == 0
    	HTEST = 0;
		for I = 1:8
      		HI = T * (AH(I,1) + BH(I,1) * T / 2 + CH(I,1) * T^2 / 3);
      		HI = 1.8 * HI;
      		HTEST = HTEST + Z(I,1) * XMW(I,1) * HI;
		end
	else
      	HTEST = 0;
		for I = 1:8 
      		HI = T * (AG(I,1) + BG(I,1) * T / 2 + CG(I,1) * T^2 / 3);
      		HI = 1.8 * HI;
      		HI = HI + AV(I,1);
      		HTEST = HTEST + Z(I,1) * XMW(I,1) * HI;
		end
    end
        if ITY == 2
         	R1 = 3.57696 / 1000000;
        	HTEST = HTEST - R1 * (T + 273.15);
    	end
		
    ERR = HTEST - H;
	
	if ITY == 0
      	DH = 0.0;
    	for I = 1:8
      		DHI = AH(I,1) + BH(I,1) * T + CH(I,1) * T^2;
      		DHI = 1.8 * DHI;
      		DH = DH + Z(I,1) * XMW(I,1) * DHI;
		end
	else
      	DH=0.0;
    	for I = 1:8
      		DHI = AG(I,1) + BG(I,1) * T + CG(I,1) * T^2;
      		DHI = 1.8 * DHI;
      		DH = DH + Z(I,1) * XMW(I,1) * DHI;
		end
    end
    
    if ITY == 2
      	R3 = 3.57696/1000000;
     	DH = DH - R3;
 	end
	
    DT = -ERR / DH;
    T = T + DT;
  	if abs(DT) < 1*10^(-12)
    	break
  	end
  	if J == 100
  		T = TIN;
  	end
end
TCR = T;

== matlab function COSTEP_Exergy/Stripper/TCC Initial Temperature in Stripper °C /MATLAB Function ==
  data: AH input; TCC output; BH input; CH input; AG input; BG input; CG input; AV input; XMW input; XLC input; ETC input; UTLC input; ITY input; TCC input
function TCC  = TempLoop(AH,BH,CH,AG,BG,CG,AV,XMW,XLC,ETC,UTLC,ITY,TCC)

ESC = ETC/UTLC;
     
Z = XLC;
T = TCC;
H = ESC;
TIN=T;

for J = 1:100
	
	if ITY == 0
    	HTEST = 0;
		for I = 1:8
      		HI = T * (AH(I,1) + BH(I,1) * T / 2 + CH(I,1) * T^2 / 3);
      		HI = 1.8 * HI;
      		HTEST = HTEST + Z(I,1) * XMW(I,1) * HI;
		end
	else
      	HTEST = 0;
		for I = 1:8 
      		HI = T * (AG(I,1) + BG(I,1) * T / 2 + CG(I,1) * T^2 / 3);
      		HI = 1.8 * HI;
      		HI = HI + AV(I,1);
      		HTEST = HTEST + Z(I,1) * XMW(I,1) * HI;
		end
    end
        if ITY == 2
         	R1 = 3.57696 / 1000000;
        	HTEST = HTEST - R1 * (T + 273.15);
    	end
		
    ERR = HTEST - H;
	
	if ITY == 0
      	DH = 0.0;
    	for I = 1:8
      		DHI = AH(I,1) + BH(I,1) * T + CH(I,1) * T^2;
      		DHI = 1.8 * DHI;
      		DH = DH + Z(I,1) * XMW(I,1) * DHI;
		end
	else
      	DH=0.0;
    	for I = 1:8
      		DHI = AG(I,1) + BG(I,1) * T + CG(I,1) * T^2;
      		DHI = 1.8 * DHI;
      		DH = DH + Z(I,1) * XMW(I,1) * DHI;
		end
    end
    
    if ITY == 2
      	R3 = 3.57696/1000000;
     	DH = DH - R3;
 	end
	
    DT = -ERR / DH;
    T = T + DT;
  	if abs(DT) < 1*10^(-12)
    	break
  	end
  	if J == 100
  		T = TIN;
  	end
end
TCC = T;

== matlab function COSTEP_Exergy/Mixing Zone/TCV Initial Temperature in Mixing zone °C /MATLAB Function ==
  data: AH input; TCV output; BH input; CH input; AG input; BG input; CG input; AV input; XMW input; XVV input; ETV input; UTVV input; ITY input; TCV input
function TCV  = TempLoop(AH,BH,CH,AG,BG,CG,AV,XMW,XVV,ETV,UTVV,ITY,TCV)

ESV = ETV/UTVV;
     
Z = XVV;
T = TCV;
H = ESV;
TIN=T;

for J = 1:100
	
	if ITY == 0
    	HTEST = 0;
		for I = 1:8
      		HI = T * (AH(I,1) + BH(I,1) * T / 2 + CH(I,1) * T^2 / 3);
      		HI = 1.8 * HI;
      		HTEST = HTEST + Z(I,1) * XMW(I,1) * HI;
		end
	else
      	HTEST = 0;
		for I = 1:8 
      		HI = T * (AG(I,1) + BG(I,1) * T / 2 + CG(I,1) * T^2 / 3);
      		HI = 1.8 * HI;
      		HI = HI + AV(I,1);
      		HTEST = HTEST + Z(I,1) * XMW(I,1) * HI;
		end
    end
        if ITY == 2
         	R1 = 3.57696 / 1000000;
        	HTEST = HTEST - R1 * (T + 273.15);
    	end
		
    ERR = HTEST - H;
	
	if ITY == 0
      	DH = 0.0;
    	for I = 1:8
      		DHI = AH(I,1) + BH(I,1) * T + CH(I,1) * T^2;
      		DHI = 1.8 * DHI;
      		DH = DH + Z(I,1) * XMW(I,1) * DHI;
		end
	else
      	DH=0.0;
    	for I = 1:8
      		DHI = AG(I,1) + BG(I,1) * T + CG(I,1) * T^2;
      		DHI = 1.8 * DHI;
      		DH = DH + Z(I,1) * XMW(I,1) * DHI;
		end
    end
    
    if ITY == 2
      	R3 = 3.57696/1000000;
     	DH = DH - R3;
 	end
	
    DT = -ERR / DH;
    T = T + DT;
  	if abs(DT) < 1*10^(-12)
    	break
  	end
  	if J == 100
  		T = TIN;
  	end
end
TCV = T;

== matlab function COSTEP_Exergy/Random number generator/MATLAB Function ==
  data: G input; G_out output
function G_out = checkG(G)
    G_out = zeros(1, 1);
    coder.extrinsic("evalin")
    % Lets first check if "G" exists in the workspace form
    % Auto_run_COSTEP.m
    ise = evalin('base', 'exist(''G'',''var'') == 1');
    if ise 
        G_out = evalin('base', 'G');
    else
        G_out = G;
    end
end
